simulink model "Blank_Model"  (R2022a)
settings: Solver=FixedStepAuto  StartTime=0.0  StopTime=500  FixedStep=0.0001  RelTol=1e-9
undefined symbols (not defined in the file): DiscIntNeverNeededParam, Serial_Port, Standard_Devices
libraries: simulink_extras x10, simulink x2, sldrtlib x2
settings Model: SimulationMode=external  Creator=zachn  LastModifiedBy=domin
settings SolverCC: AlgebraicLoopSolver=TrustRegion
settings DataIOCC: SaveFormat=StructureWithTime  InspectSignalLogs=on
settings DebuggingCC: UnconnectedInputMsg=warning  UnconnectedOutputMsg=warning  UnconnectedLineMsg=warning  SFMachineParentedDataDiag=warning
settings HardwareCC: ProdBitPerLong=64  ProdHWDeviceType=Intel->x86-64 (Linux 64)
settings RTWCC: Description=Simulink Desktop Real-Time  SystemTargetFile=sldrt.tlc  TemplateMakefile=sldrt.tmf  RTWCompilerOptimization=on  DLArmComputeVersion=19.05
settings CodeAppCC: MaxIdLength=95
settings SimulinkDesktopRealTimeCC: TargetLibSuffix=_sldrt.a  TargetPreCompLibLocation=C:\Program Files\MATLAB\R2022a\toolbox\sldrt\lib\win64

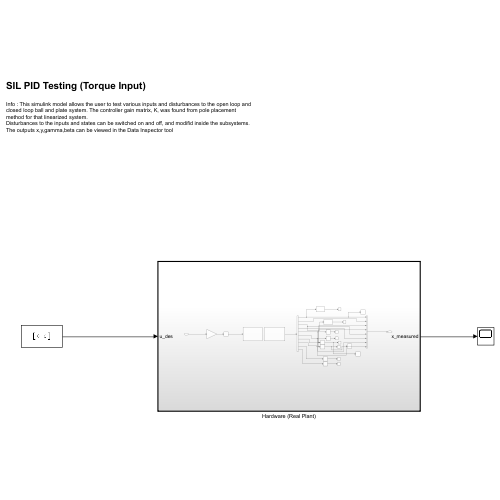
[thumbnail: Simulink's stored preview of the top-level diagram]
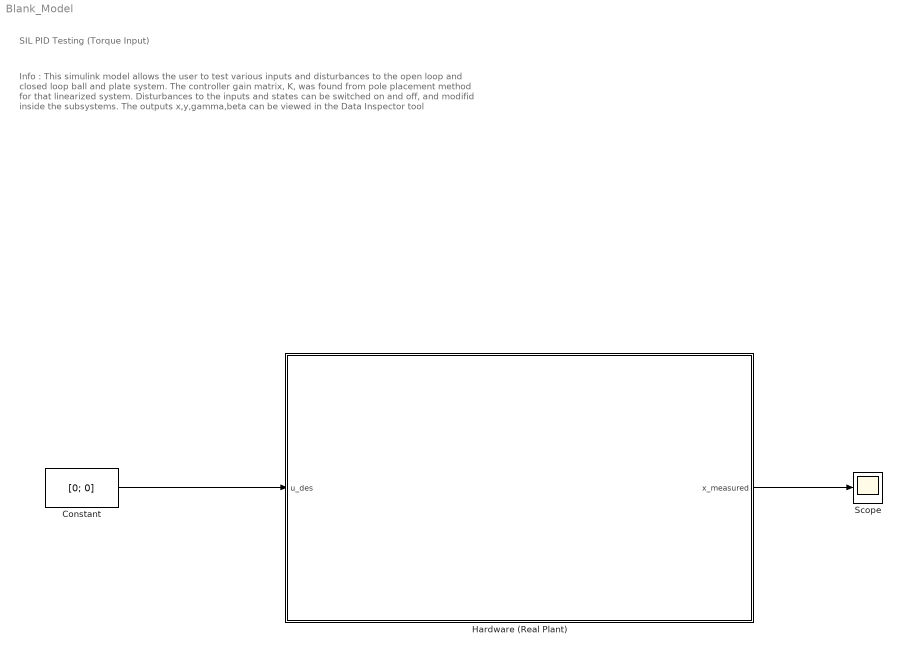
== system Blank_Model ==
  note: Info : This simulink model allows the user to test various inputs and disturbances to the open loop and closed loop ball and plate system. The controller gain matrix, K, was found from pole placement
      | method for that linearized system.
      | Disturbances to the inputs and states can be switched on and off, and modifid inside the subsystems.
      | The outputs x,y,gamma,beta can be viewed in the Data Inspector tool
  note: SIL PID Testing (Torque Input)
  Constant : Constant  Value=[0; 0]
  Hardware (Real Plant) : Subsystem  TreatAsAtomicUnit=on
  Scope : Scope
  wires:
  Constant/1 -> Hardware (Real Plant)/1(u_des)
  Hardware (Real Plant)/1(x_measured) -> Scope/1

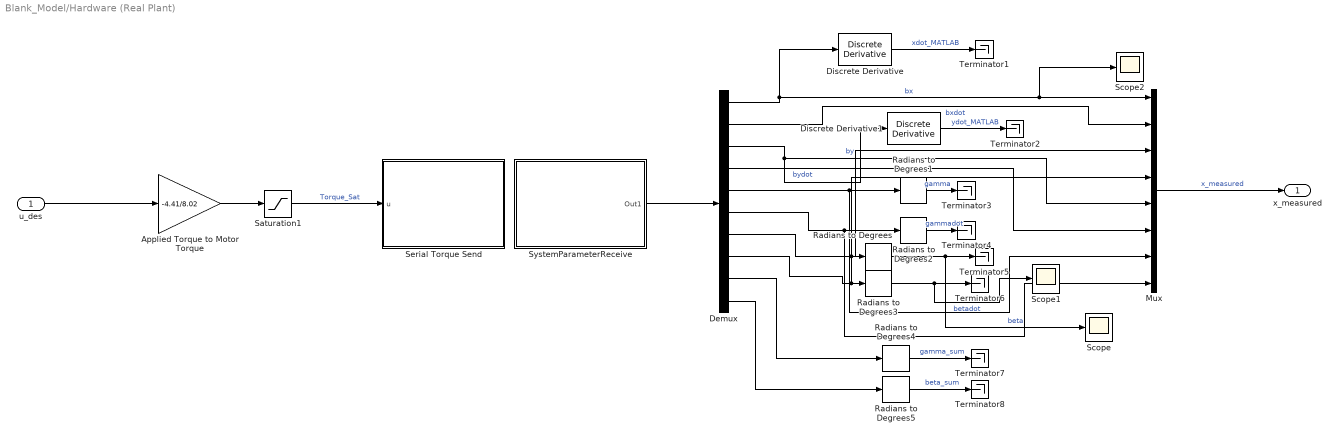
== system Blank_Model/Hardware (Real Plant) ==
  u_des : Inport
  Applied Torque to Motor Torque : Gain  Gain=-4.41/8.02
  Demux : Demux  Outputs=10
  Discrete Derivative : simulink/Discrete/Discrete Derivative  gainval=1.0  ICPrevScaledInput=0.0  OutMin=[]  OutMax=[]  OutDataType=fixdt(1, 16)  OutScaling=2^-10  DoSatur=off
  Discrete Derivative1 : simulink/Discrete/Discrete Derivative  gainval=1.0  ICPrevScaledInput=0.0  OutMin=[]  OutMax=[]  OutDataType=fixdt(1, 16)  OutScaling=2^-10  DoSatur=off
  Mux : Mux  Inputs=8
  Radians to Degrees{,1..5} (6 alike) : simulink_extras/Transformations/Radians to Degrees
  Saturation1 : Saturate  UpperLimit=1  LowerLimit=-1
  Scope : Scope
  Scope1 : Scope
  Scope2 : Scope
  Serial Torque Send : Subsystem
  SystemParameterReceive : Subsystem
  Terminator{1..8} (8 alike) : Terminator
  x_measured : Outport
  wires:
  u_des/1 -> Applied Torque to Motor Torque/1
  Applied Torque to Motor Torque/1 -> Saturation1/1
  Saturation1/1 -> Serial Torque Send/1(u)  "Torque_Sat"
  Discrete Derivative1/1 -> Terminator2/1  "ydot_MATLAB"
  Demux/3 -> Mux/5, Discrete Derivative1/1  "by"
  Radians to Degrees5/1 -> Terminator8/1  "beta_sum"
  Demux/9 -> Radians to Degrees4/1
  Discrete Derivative/1 -> Terminator1/1  "xdot_MATLAB"
  SystemParameterReceive/1(Out1) -> Demux/1
  Demux/1 -> Discrete Derivative/1, Scope2/1, Mux/1  "bx"
  Demux/8 -> Mux/4, Radians to Degrees3/1
  Radians to Degrees4/1 -> Terminator7/1  "gamma_sum"
  Radians to Degrees2/1 -> Terminator4/1  "gammadot"
  Radians to Degrees3/1 -> Scope1/1, Terminator6/1  "betadot"
  Demux/4 -> Mux/6  "bydot"
  Demux/6 -> Mux/8, Radians to Degrees2/1
  Demux/5 -> Mux/7, Radians to Degrees1/1
  Demux/7 -> Mux/3, Radians to Degrees/1
  Radians to Degrees/1 -> Scope/1, Terminator5/1  "beta"
  Demux/10 -> Radians to Degrees5/1
  Demux/2 -> Mux/2  "bxdot"
  Mux/1 -> x_measured/1  "x_measured"
  Radians to Degrees1/1 -> Terminator3/1  "gamma"

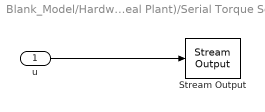
== system Blank_Model/Hardware (Real Plant)/Serial Torque Send ==
  u : Inport
  Stream Output : sldrtlib/Stream Output  SampleTime=0.005  MaxMissedTicks=10  ShowMissedTicks=off  YieldWhenWaiting=off  DrvName=Standard_Devices/Serial_Port  DrvAddress=6  DrvOptions=[115200 8 0 0 1 0 0 0]  PortSizes=2  FormatString='%g %g\n'  ShowReady=off  ShowError=off  InitialValue=[]  FinalValue=[]
      settings: AttributesFormatString=Serial Port [6]  SourceProductBaseCode=WT
  wires:
  u/1 -> Stream Output/1

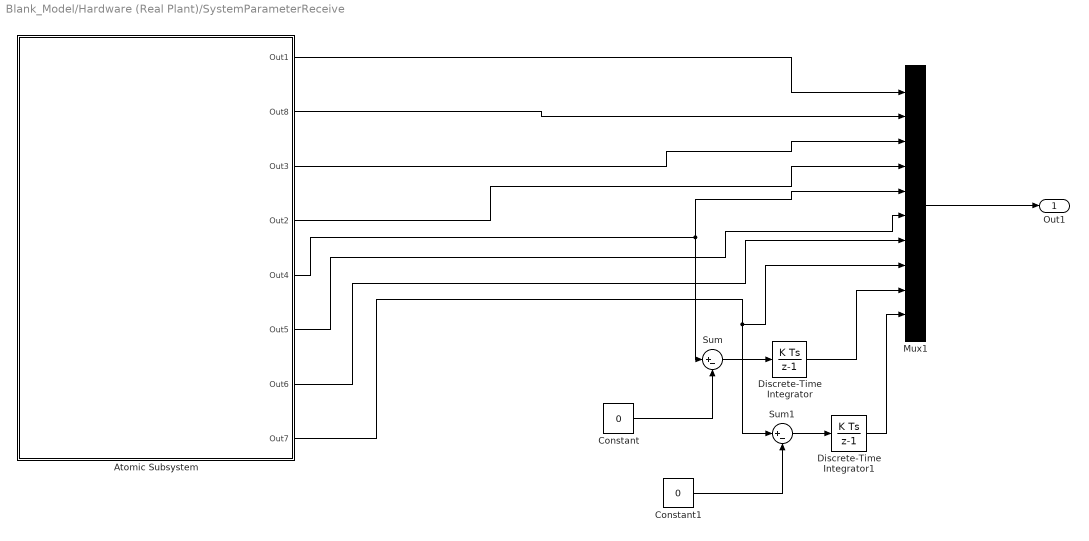
== system Blank_Model/Hardware (Real Plant)/SystemParameterReceive ==
  Atomic Subsystem : Subsystem  TreatAsAtomicUnit=on
  Constant : Constant  Value=0
  Constant1 : Constant  Value=0
  Discrete-Time Integrator : DiscreteIntegrator  SampleTime=-1  ICPrevOutput=DiscIntNeverNeededParam  ICPrevScaledInput=DiscIntNeverNeededParam
  Discrete-Time Integrator1 : DiscreteIntegrator  SampleTime=-1  ICPrevOutput=DiscIntNeverNeededParam  ICPrevScaledInput=DiscIntNeverNeededParam
  Mux1 : Mux  Inputs=10
  Sum : Sum  Inputs=|+-
  Sum1 : Sum  Inputs=|+-
  Out1 : Outport
  wires:
  Atomic Subsystem/3(Out3) -> Mux1/3
  Atomic Subsystem/7(Out6) -> Mux1/7
  Atomic Subsystem/8(Out7) -> Sum1/1, Mux1/8
  Mux1/1 -> Out1/1
  Atomic Subsystem/5(Out4) -> Sum/1, Mux1/5
  Atomic Subsystem/4(Out2) -> Mux1/4
  Atomic Subsystem/2(Out8) -> Mux1/2
  Atomic Subsystem/1(Out1) -> Mux1/1
  Constant/1 -> Sum/2
  Sum/1 -> Discrete-Time Integrator/1
  Discrete-Time Integrator/1 -> Mux1/9
  Constant1/1 -> Sum1/2
  Sum1/1 -> Discrete-Time Integrator1/1
  Atomic Subsystem/6(Out5) -> Mux1/6
  Discrete-Time Integrator1/1 -> Mux1/10

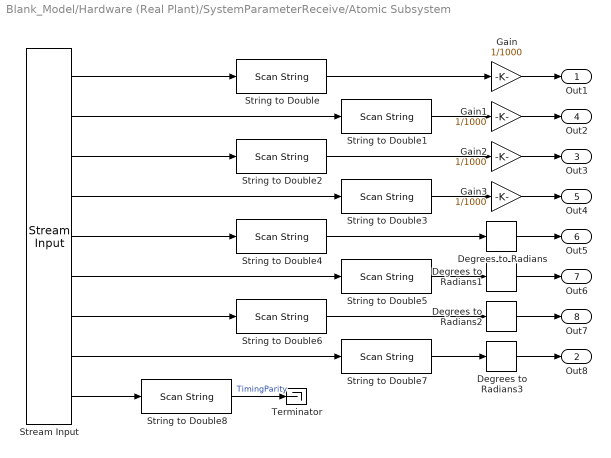
== system Blank_Model/Hardware (Real Plant)/SystemParameterReceive/Atomic Subsystem ==
  Degrees to Radians{,1..3} (4 alike) : simulink_extras/Transformations/Degrees to Radians
  Gain{,1..3} (4 alike) : Gain  Gain=1/1000  OutDataTypeStr=double
  Stream Input : sldrtlib/Stream Input  SampleTime=0.005  MaxMissedTicks=10  ShowMissedTicks=off  YieldWhenWaiting=on  DrvName=Standard_Devices/Serial_Port  DrvAddress=6  DrvOptions=[115200 8 0 0 1 0 0 0]  DataTypes={'string','string','string','string','string','string','string','string','string'}  FormatString='%s %s %s %s %s %s %s %s %s'  Terminator={'\r', '\n'}  ShowReady=off  ShowError=off
      settings: AttributesFormatString=Serial Port [6]  SourceProductBaseCode=WT
  String to Double : ScanString  Format="\"%d\""
  String to Double{1..8} (8 alike) : ScanString  Format="\"%lf\""
  Terminator : Terminator
  Out1 : Outport
  Out8 : Outport  Port=2
  Out3 : Outport  Port=3
  Out2 : Outport  Port=4
  Out4 : Outport  Port=5
  Out5 : Outport  Port=6
  Out6 : Outport  Port=7
  Out7 : Outport  Port=8
  wires:
  String to Double5/1 -> Degrees to Radians1/1
  String to Double4/1 -> Degrees to Radians/1
  String to Double1/1 -> Gain1/1
  Stream Input/8 -> String to Double7/1
  Stream Input/9 -> String to Double8/1
  Stream Input/5 -> String to Double4/1
  String to Double2/1 -> Gain2/1
  Stream Input/3 -> String to Double2/1
  String to Double/1 -> Gain/1
  Stream Input/1 -> String to Double/1
  Stream Input/4 -> String to Double3/1
  String to Double7/1 -> Degrees to Radians3/1
  Stream Input/2 -> String to Double1/1
  String to Double8/1 -> Terminator/1  "TimingParity"
  String to Double6/1 -> Degrees to Radians2/1
  Stream Input/7 -> String to Double6/1
  String to Double3/1 -> Gain3/1
  Stream Input/6 -> String to Double5/1
  Gain/1 -> Out1/1
  Gain1/1 -> Out2/1
  Gain2/1 -> Out3/1
  Gain3/1 -> Out4/1
  Degrees to Radians/1 -> Out5/1
  Degrees to Radians1/1 -> Out6/1
  Degrees to Radians2/1 -> Out7/1
  Degrees to Radians3/1 -> Out8/1
